simulink model "untitled"  (R2016a)
settings: Solver=VariableStepAuto  StartTime=0.0  StopTime=60e-3  RelTol=1e-3
libraries: powerlib x13
settings Model: Creator=VARUN SINGH  LastModifiedBy=VARUN SINGH

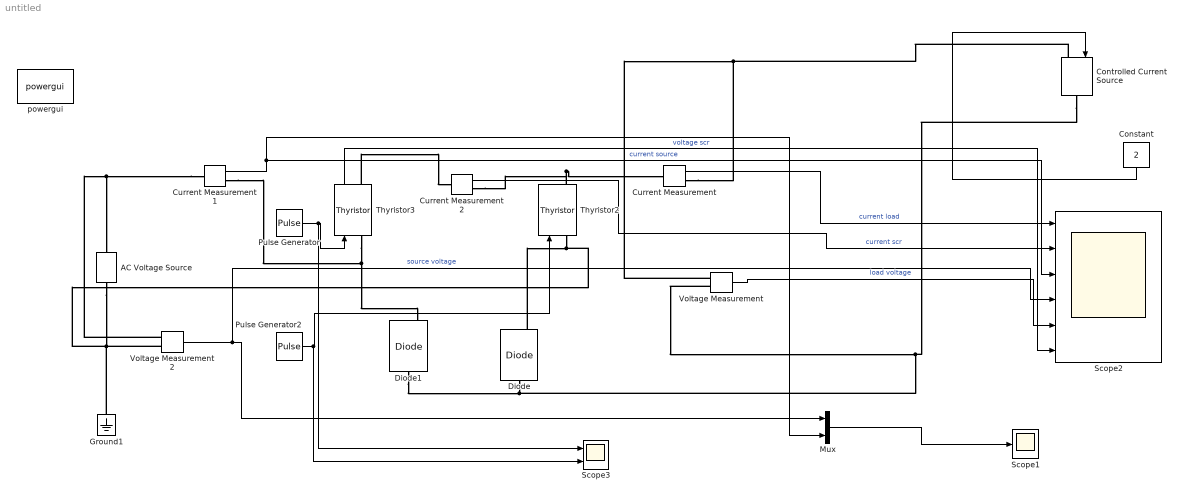
== system untitled ==
  AC Voltage Source : powerlib/Electrical Sources/AC Voltage Source  Amplitude=220  Phase=0  Frequency=50  SampleTime=0  Measurements=None  BusType=swing  Pref=10e3  Qref=0  Qmin=-inf  Qmax=+inf
  Constant : Constant  Value=2
  Controlled Current Source : powerlib/Electrical Sources/Controlled Current Source  Initialize=on  Source_Type=AC  Amplitude=2  Phase=0  Frequency=0  Measurements=None
  Current Measurement : powerlib/Measurements/Current Measurement  PhasorSimulation=off  OutputType=Complex  PSBequivalent=0
  Current Measurement1 : powerlib/Measurements/Current Measurement  PhasorSimulation=off  OutputType=Complex  PSBequivalent=0
  Current Measurement2 : powerlib/Measurements/Current Measurement  PhasorSimulation=off  OutputType=Complex  PSBequivalent=0
  Diode : powerlib/Power Electronics/Diode  Ron=0.001  Lon=0  Vf=0.8  IC=0  UseSnubber=off  Rs=500  Cs=250e-9  Measurements=on
  Diode1 : powerlib/Power Electronics/Diode  Ron=0.001  Lon=0  Vf=0.8  IC=0  UseSnubber=off  Rs=500  Cs=250e-9  Measurements=on
  Ground1 : powerlib/Elements/Ground  LConnTagsString=a
  Mux : Mux  Inputs=2
  Pulse Generator : DiscretePulseGenerator  PulseType=Time based  Period=20e-3  PulseWidth=5  PhaseDelay=(20e-3/360)*60
  Pulse Generator2 : DiscretePulseGenerator  PulseType=Time based  Period=20e-3  PulseWidth=5  PhaseDelay=10e-3+((20e-3/360)*60)
  Scope1 : Scope
  Scope2 : Scope  NumInputPorts=6
  Scope3 : Scope  NumInputPorts=2
  Thyristor2 : powerlib/Power Electronics/Thyristor  Ron=0.001  Lon=0  Vf=0.8  IC=0  Rs=500  Cs=250e-9  Measurements=on
  Thyristor3 : powerlib/Power Electronics/Thyristor  Ron=0.001  Lon=0  Vf=0.8  IC=0  Rs=500  Cs=250e-9  Measurements=on
  Voltage Measurement : powerlib/Measurements/Voltage Measurement  PhasorSimulation=off  OutputType=Complex  PSBequivalent=0
  Voltage Measurement2 : powerlib/Measurements/Voltage Measurement  PhasorSimulation=off  OutputType=Complex  PSBequivalent=0
  powergui : powerlib/powergui  Priority=1  SimulationMode=Continuous  SolverType=Tustin/Backward Euler (TBE)  SampleTime=50e-6  frequency=60  SPID=off  DisableSnubberDevices=off  DisableRonSwitches=off  DisableVfSwitches=off  SwTol=0  DisplayEquations=off  Interpol=off  ExternalGateDelay=off  methode=off  Ts=10  FunctionMessages=off  echomessages=off  HookPort=off  EnableUseOfTLC=off  x0status=blocks  frequencyindice=50  Pbase=100e6  ErrMax=1e-4  Iterations=50  UnitsV=kV  UnitsW=MW  buscounter=0  RestoreLinks=warning  ResistiveCurrentMeasurement=off  Frange=[0:2:500]  Ylog=off  Xlog=on  ShowGrid=off  save=off  variable=ZData  structure=0  ZoomFFT=off  StartTime=0.0  cycles=1  DisplayStyle=1  fundamental=60  FreqAxis=off  MaxFrequency=1000  frequencyindicesteady=1  RmsSteady=1  display=off
  wires:
  Pulse Generator/1 -> Scope3/1, Thyristor3/1
  Pulse Generator2/1 -> Scope3/2, Thyristor2/1
  Current Measurement1/1 -> Mux/2, Scope2/3  "current source"
  Voltage Measurement/1 -> Scope2/5  "load voltage"
  Voltage Measurement2/1 -> Mux/1, Scope2/4  "source voltage"
  Thyristor3/1 -> Scope2/6  "voltage scr"
  Current Measurement/1 -> Scope2/1  "current load"
  Current Measurement2/1 -> Scope2/2  "current scr"
  Mux/1 -> Scope1/1
  Constant/1 -> Controlled Current Source/1
  connections:
  Thyristor3/LConn1 -- Diode1/RConn1 -- Current Measurement1/RConn1
  Thyristor2/LConn1 -- AC Voltage Source/LConn1 -- Ground1/LConn1 -- Voltage Measurement2/LConn2 -- Diode/RConn1
  Controlled Current Source/RConn1 -- Voltage Measurement/LConn2 -- Diode1/LConn1 -- Diode/LConn1
  Thyristor2/RConn1 -- Current Measurement2/RConn1 -- Current Measurement/LConn1
  Current Measurement1/LConn1 -- Voltage Measurement2/LConn1 -- AC Voltage Source/RConn1
  Current Measurement/RConn1 -- Controlled Current Source/LConn1 -- Voltage Measurement/LConn1
  Thyristor3/RConn1 -- Current Measurement2/LConn1
